simulink model "Ramp_Signal"  (R2023a)
settings: Solver=VariableStepAuto  StartTime=0.0  StopTime=10.0  RelTol=1e-3
libraries: simulink x1
settings Model: Creator=Aman  LastModifiedBy=Aman

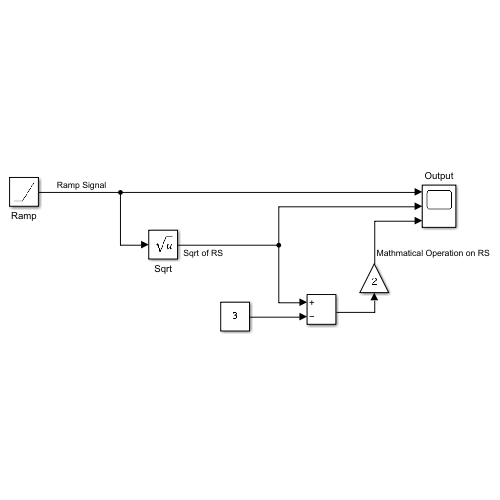
[thumbnail: Simulink's stored preview of the top-level diagram]
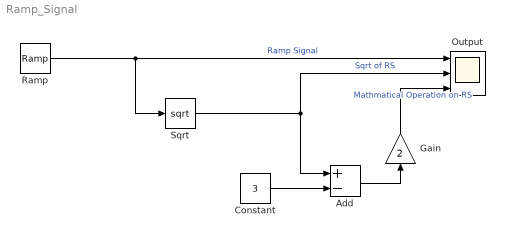
== system Ramp_Signal ==
  Add : Sum  Inputs=+-
  Constant : Constant  Value=3
  Gain : Gain  Gain=2
  Output : Scope  NumInputPorts=3
  Ramp : simulink/Sources/Ramp  slope=1  start=0  InitialOutput=0
  Sqrt : Sqrt
  wires:
  Ramp/1 -> Sqrt/1, Output/1  "Ramp Signal"
  Sqrt/1 -> Add/1, Output/2  "Sqrt of RS"
  Constant/1 -> Add/2
  Add/1 -> Gain/1
  Gain/1 -> Output/3  "Mathmatical Operation on RS"
